simulink model "test"  (R2019b)
settings: Solver=VariableStepAuto  StartTime=0.0  StopTime=10.0  RelTol=1e-3
settings Model: Creator=yangy  LastModifiedBy=yangy
settings SFSimCC: CustomCodeUndefinedFunction=UseInterfaceOnly

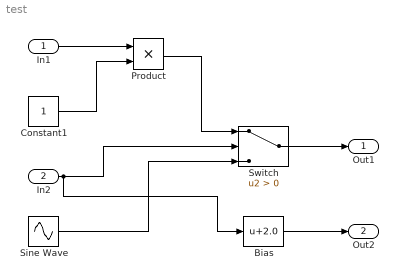
== system test ==
  In1 : Inport
  In2 : Inport  Port=2
  Bias : Bias  Bias=2.0
  Constant1 : Constant
  Product : Product
  Sine Wave : Sin  SampleTime=0
  Switch : Switch  Criteria=u2 > Threshold
  Out1 : Outport  VectorParamsAs1DForOutWhenUnconnected=off
  Out2 : Outport  Port=2  VectorParamsAs1DForOutWhenUnconnected=off
  wires:
  Constant1/1 -> Product/2
  Product/1 -> Switch/1
  Sine Wave/1 -> Switch/3
  In2/1 -> Bias/1, Switch/2
  Switch/1 -> Out1/1
  In1/1 -> Product/1
  Bias/1 -> Out2/1
